simulink model "lab5_ASP_DavydovA"  (R2022b)
settings: Solver=VariableStepAuto  StartTime=0.0  StopTime=10.0  RelTol=1e-3
libraries: matrix_library x2, audiosources x1, dspvision x1, dspfdesign x1
settings Model: Creator=FASER  LastModifiedBy=FASER

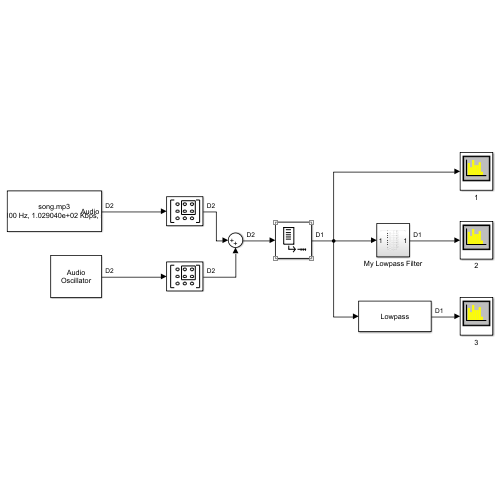
[thumbnail: Simulink's stored preview of the top-level diagram]
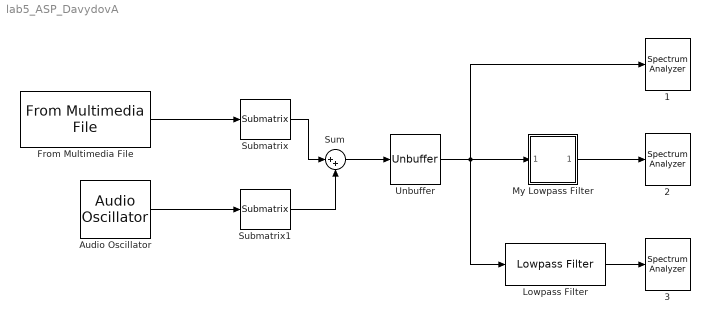
== system lab5_ASP_DavydovA ==
  1 : SpectrumAnalyzer
  2 : SpectrumAnalyzer
  3 : SpectrumAnalyzer
  Audio Oscillator : audiosources/Audio Oscillator  FrequencyPort=off  Frequency=17000  AmplitudePort=off  Amplitude=1  DCOffsetPort=off  PhaseOffset=0  DCOffset=0  WidthPort=off  Width=1  DutyCyclePort=off  DutyCycle=0.5  SampsPerFrame=1024  Fs=44100  OutputDataType=double  SimulateUsing=Code generation
      settings: SignalType=sine
  From Multimedia File : dspvision/From Multimedia File  inputFilename=C:\Users\FASER\Documents\MATLAB\Lab_5\song.mp3  readRange=[1 Inf]  loop=on  numPlays=inf  outputStreams=Audio only  videoDataType=single  audioDataType=double  inheritSampleTime=on  userDefinedSampleTime=1/30  noAudioOutput=off  isIntensityVideo=off  fourcc=RGB  colorVideoFormat=Separate color signals  outputEOF=off  dataOrg=Column-major  audioFrameSize=1024  computeAudioFrameSize=off  outSamplingMode=Sample based
      settings: LibrarySourceBlock=audiosources/From Multimedia File
  Lowpass Filter : dspfdesign/Lowpass Filter  FilterType=FIR  DesignForMinimumOrder=on  FilterOrder=50  PassbandFrequency=8e3  StopbandFrequency=12e3  PassbandRipple=0.1  StopbandAttenuation=80  InheritSampleRate=off  SampleRate=44100  SimulateUsing=Interpreted execution  roundingMode=Floor  coeffsDataTypeStr=fixdt(1,16)
  My Lowpass Filter : Subsystem
  Submatrix : matrix_library/Submatrix  RowSpan=Range of rows  RowStartMode=First  RowStartIndex=1  RowEndMode=Last  RowEndIndex=1  ColSpan=One column  ColStartMode=First  ColStartIndex=1  ColEndMode=Last  ColEndIndex=1
  Submatrix1 : matrix_library/Submatrix  RowSpan=Range of rows  RowStartMode=First  RowStartIndex=1  RowEndMode=Last  RowEndIndex=1  ColSpan=One column  ColStartMode=First  ColStartIndex=1  ColEndMode=Last  ColEndIndex=1
  Sum : Sum  Inputs=|++
  Unbuffer : Unbuffer
  wires:
  From Multimedia File/1 -> Submatrix/1
  Audio Oscillator/1 -> Submatrix1/1
  Submatrix/1 -> Sum/1
  Submatrix1/1 -> Sum/2
  Sum/1 -> Unbuffer/1
  Unbuffer/1 -> Lowpass Filter/1, My Lowpass Filter/1(Input), 1/1
  My Lowpass Filter/1(Output) -> 2/1
  Lowpass Filter/1 -> 3/1

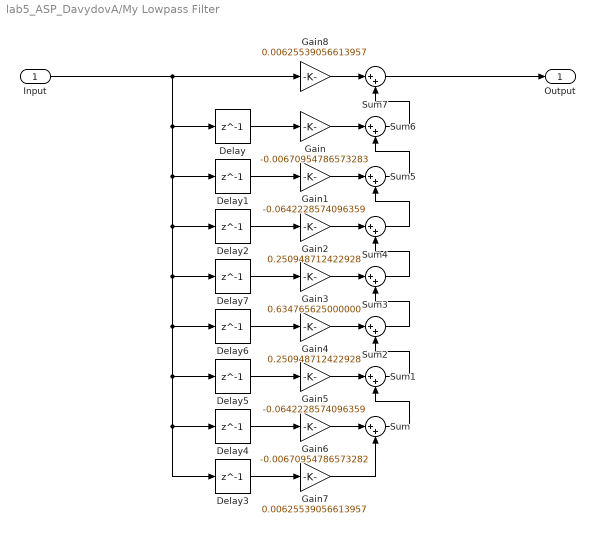
== system lab5_ASP_DavydovA/My Lowpass Filter ==
  Input : Inport
  Delay{,1..7} (8 alike) : Delay  DelayLength=1
  Gain : Gain  Gain=-0.00670954786573283
  Gain1 : Gain  Gain=-0.0642228574096359
  Gain2 : Gain  Gain=0.250948712422928
  Gain3 : Gain  Gain=0.634765625000000
  Gain4 : Gain  Gain=0.250948712422928
  Gain5 : Gain  Gain=-0.0642228574096359
  Gain6 : Gain  Gain=-0.00670954786573282
  Gain7 : Gain  Gain=0.00625539056613957
  Gain8 : Gain  Gain=0.00625539056613957
  Sum{,1..7} (8 alike) : Sum  Inputs=|++
  Output : Outport
  wires:
  Sum5/1 -> Sum6/2
  Gain1/1 -> Sum5/1
  Delay6/1 -> Gain4/1
  Sum1/1 -> Sum2/2
  Delay2/1 -> Gain2/1
  Gain6/1 -> Sum/1
  Gain8/1 -> Sum7/1
  Gain4/1 -> Sum2/1
  Input/1 -> Delay/1, Delay1/1, Delay2/1, Delay7/1, Delay6/1, Delay5/1, Delay3/1, Delay4/1, Gain8/1
  Delay/1 -> Gain/1
  Sum/1 -> Sum1/2
  Sum6/1 -> Sum7/2
  Delay4/1 -> Gain6/1
  Gain7/1 -> Sum/2
  Delay5/1 -> Gain5/1
  Gain5/1 -> Sum1/1
  Sum7/1 -> Output/1
  Sum3/1 -> Sum4/2
  Delay7/1 -> Gain3/1
  Gain2/1 -> Sum4/1
  Gain3/1 -> Sum3/1
  Sum2/1 -> Sum3/2
  Delay1/1 -> Gain1/1
  Delay3/1 -> Gain7/1
  Sum4/1 -> Sum5/2
  Gain/1 -> Sum6/1
